simulink model "KD_cl_harness_forthao"  (R2015a)
settings: Solver=ode45  StartTime=0  StopTime=50  FixedStep=0.01  MaxStep=0.005  RelTol=1e-4  AbsTol=1e-4
InitFcn:
  | load KD_const_coeffs_0624
  | load pexhat_stuff
  | load expcon
  | load thr_ff_map
values from neighbouring files (symbols this model uses):
  c_0 = 0    [expcon.mat]
  c_1 = 1    [expcon.mat]
  c_100 = 100    [expcon.mat]
  c_1000 = 1000    [expcon.mat]
  c_10000 = 10000    [expcon.mat]
  c_1000inv = 0.0010000000475    [expcon.mat]    (also in pexhat_stuff.mat)
  c_100inv = 0.00999999977648    [expcon.mat]
  c_1_int = 1    [expcon.mat]
  c_1d2p4 = 0.416666656733    [expcon.mat]
  c_1p7 = 1.70000004768    [expcon.mat]
  c_4400inv = 0.000227272728807    [pexhat_stuff.mat]
  c_5500inv = 0.000181818177225    [expcon.mat]
  c_80 = 80    [expcon.mat]
  c_90 = 90    [expcon.mat]
  c_cal_phi = 7.6395999713e-06    [expcon.mat]
  c_compmap = [28125.0058594 29577.4082031 31350.1035156 33776.21875 37051.9296875 41026.2695312 45453.9960938 50160.3515625 55029.671875 59986.109375 64980.4296875 69980.4375 ... (320 elements, 20x16)]    [expcon.mat]
  c_ctok = 273.149993896    [expcon.mat]
  c_fflow_max = inf    [expcon.mat]
  c_fflow_min = 0    [expcon.mat]
  c_filt = 0.949999988079    [expcon.mat]
  c_flowdiv = 9.99999974738e-05    [expcon.mat]
  c_flowmin = 0    [expcon.mat]
  c_flowmult = 10000    [expcon.mat]
  c_inf = inf    [expcon.mat]
  c_km1d2k = 0.142857149243    [expcon.mat]
  c_mm3tokgpers = 2.77333338516e-08    [expcon.mat]
  c_n1 = -1    [expcon.mat]
  c_p00001 = 9.99999974738e-06    [expcon.mat]
  c_p01 = 0.00999999977648    [pexhat_stuff.mat]
  c_p016 = 0.01600000076    [expcon.mat]
  c_p1429 = 0.142900004983    [expcon.mat]
  c_p1e9 = 9.99999971718e-10    [expcon.mat]
  c_p4167 = 0.416700005531    [expcon.mat]    (also in pexhat_stuff.mat = 0.416666656733)
  c_p4d1p4 = 0.285714298487    [expcon.mat]
  c_p5401 = 0.540099978447    [expcon.mat]
  c_p9 = 0.899999976158    [expcon.mat]
  c_pincomp = 97.4216003418    [expcon.mat]
  c_ra = 287.002807617    [expcon.mat]
  c_rair = 287.09979248    [expcon.mat]
  c_Rby1000 = 0.000287000002572    [expcon.mat]
  c_roacorr = 8.05689978733e-06    [expcon.mat]
  c_rpmtoradpers = 0.104719758034    [expcon.mat]
  c_svrthrottle1 = [0.924875080585 0.575991511345 0.0858279466629 0.820202827454 0.445821881294 0.509882986546 0.0428557097912 0.753634572029 0]    [expcon.mat]
  c_svrthrottle2 = [0.145454958081 0.14545533061 0.363636374474 0.509091556072 0.509090721607 0.509091317654 0.545454084873 0.618182241917 0.145454272628]    [expcon.mat]
  c_svrthrottlearg = 0.10000000149    [expcon.mat]
  c_svrthrottlebeta = [2282.12670898 -3239.46044922 -142.784469604 -2660.34570312 1434.34350586 4150.43994141 -1580.68164062 -1039.89575195 791.34588623]    [expcon.mat]
  c_ta_max = inf    [expcon.mat]
  c_ta_min = 270    [expcon.mat]
  c_V = 0.0077999997884    [expcon.mat]
  c_vnliftmax = 90    [expcon.mat]
  c_vnliftmin = 40    [expcon.mat]
  Coefs =     [KD_const_coeffs_0624.mat]    (also in pexhat_stuff.mat)
  const =     [KD_const_coeffs_0624.mat]    (also in pexhat_stuff.mat)
  const_exhat =     [pexhat_stuff.mat]
  eegr_map =     [expcon.mat]
  egrr_delay_init = 0    [expcon.mat]
  epim_map =     [expcon.mat]
  eplufin_ff_map =     [expcon.mat]
  expcon =     [expcon.mat]
  invta = [5 5 5 5 2.5 0 0 0 0 0 0 0 ... (240 elements, 16x15)]    [expcon.mat]
  invtacols = [1000 1200 1400 1600 1800 2000 2200 2400 2600 2800 3000 3200 ... (16 elements, 1x16)]    [expcon.mat]
  IV =     [KD_const_coeffs_0624.mat]    (also in pexhat_stuff.mat)
  Lobs_init = [0 0 0]    [expcon.mat]
  map_delay_init = 120    [expcon.mat]
  maxA_t = [51.4567184448 53.8593139648 56.3063011169 58.7576789856 61.1701469421 63.4982337952 65.6955718994 67.7161483765 69.5156555176 71.0527648926 72.2902603149 73.1961746216 ... (16 elements, 1x16)]    [expcon.mat]
  obsA = [0.985195398331  0  0; -0.188821405172  1  0; 0.000342977960827  0  1]    [expcon.mat]
  sample_time = 0.016    [expcon.mat]    (also in pexhat_stuff.mat)
  SVR_EGR =     [KD_const_coeffs_0624.mat]    (also in pexhat_stuff.mat)
  SVR_EGR_exhat =     [pexhat_stuff.mat]
  SVR_throttle =     [KD_const_coeffs_0624.mat]    (also in pexhat_stuff.mat)
  uz_init = [0 0]    [expcon.mat]
undefined symbols (not defined in the file or in its folder): k1_table, k2_table, maxL, minL, Newton, Raphson
libraries: simulink x5
(part 1 of 6)
settings Model: CovSFcnEnable=off  Creator=spolavarapu  LastModifiedBy=258242
settings SolverCC: ZeroCrossControl=DisableAll
settings DataIOCC: LimitDataPoints=off  SaveFormat=StructureWithTime  SignalLoggingSaveFormat=ModelDataLogs  SaveState=on  DSMLogging=off
settings OptimizationCC: BlockReduction=off  OptimizeBlockIOStorage=off  BufferReuse=off  GlobalBufferReuse=off  ExpressionFolding=off  ExpressionDepthLimit=2147483647  LocalBlockOutputs=off  EfficientFloat2IntCast=on  OptimizeModelRefInitCode=on
settings DebuggingCC: SignalInfNanChecking=error  SignalRangeChecking=error  ReadBeforeWriteMsg=DisableAll  WriteAfterWriteMsg=DisableAll  WriteAfterReadMsg=DisableAll  AlgebraicLoopMsg=error  ArtificialAlgebraicLoopMsg=error  SaveWithDisabledLinksMsg=error  SaveWithParameterizedLinksMsg=error  UnderspecifiedInitializationDetection=Classic  MergeDetectMultiDrivingBlocksExec=none  CheckExecutionContextPreStartOutputMsg=on  CheckExecutionContextRuntimeOutputMsg=on  BlockPriorityViolationMsg=error  SolverPrmCheckMsg=error  InheritedTsInSrcMsg=error  DiscreteInheritContinuousMsg=error  MultiTaskDSMMsg=none  SigSpecEnsureSampleTimeMsg=error  CheckMatrixSingularityMsg=error  IntegerOverflowMsg=error  ParameterUnderflowMsg=error  ParameterPrecisionLossMsg=error  ParameterTunabilityLossMsg=error  UnderSpecifiedDataTypeMsg=warning  UnnecessaryDatatypeConvMsg=warning  VectorMatrixConversionMsg=error  FcnCallInpInsideContextMsg=EnableAllAsWarning  SignalLabelMismatchMsg=warning  UnconnectedInputMsg=error  UnconnectedOutputMsg=error  UnconnectedLineMsg=error  SFcnCompatibilityMsg=error  UniqueDataStoreMsg=error  BusObjectLabelMismatch=error  RootOutportRequireBusObject=error  AssertControl=DisableAll  ModelReferenceIOMsg=error  ModelReferenceIOMismatchMessage=error  UnknownTsInhSupMsg=error  ModelReferenceDataLoggingMessage=error  StateNameClashWarn=warning  StrictBusMsg=ErrorOnBusTreatedAsVector  IntegerSaturationMsg=error
settings RTWCC: SystemTargetFile=ert.tlc  TemplateMakefile=ert_default_tmf  Description=Real-Time Workshop Embedded Coder
settings CodeAppCC: ForceParamTrailComments=on  IgnoreCustomStorageClasses=off  MangleLength=4  CustomSymbolStrType=$N$R$M  InternalIdentifier=Classic  ReqsInCode=on
settings ERTTargetCC: ParMdlRefBuildCompliant=on  CompOptLevelCompliant=on  ConcurrentExecutionCompliant=on  IncludeMdlTerminateFcn=off  GeneratePreprocessorConditionals=Disable all  SuppressErrorStatus=on  ERTFirstTimeCompliant=on  SupportAbsoluteTime=off  SupportNonFinite=off  SupportContinuousTime=off  SupportVariableSizeSignals=off  ParenthesesLevel=Maximum  ModelStepFunctionPrototypeControlCompliant=on  CPPClassGenCompliant=on  InlinedParameterPlacement=Hierarchical  ERTCustomFileTemplate=example_file_process.tlc  PreserveExpressionOrder=on  PreserveIfCondition=on

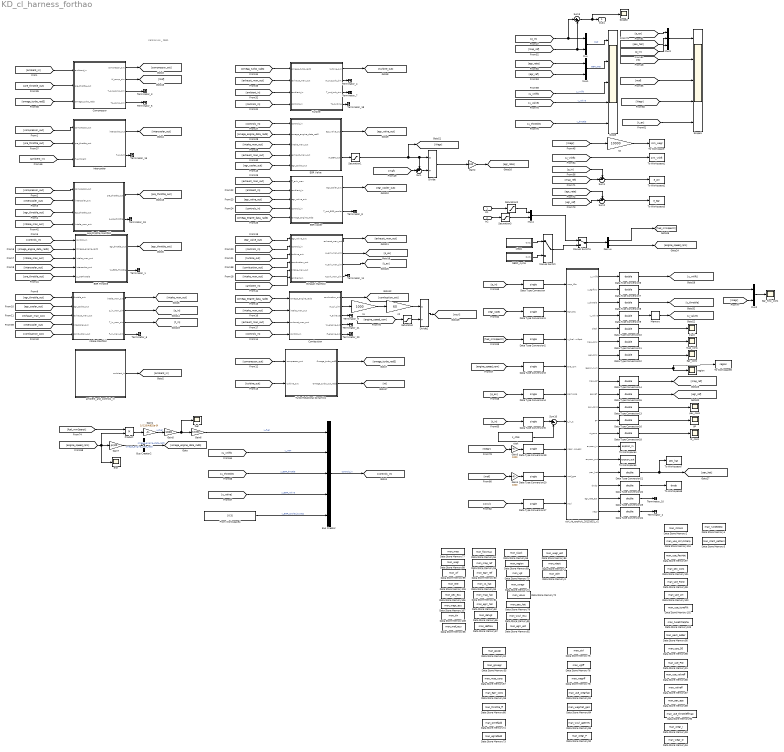
== system KD_cl_harness_forthao ==
  note: Version A4 _ 0611
  In1 : Inport  Interpolate=off
  In2 : Inport  Port=2  Interpolate=off
  Bus Creator : BusCreator  Inputs=5
  Bus Creator2 : BusCreator  Inputs=1
  Combsution : Subsystem
  Compressor : Subsystem
  Data Store Memory1 : DataStoreMemory  DataStoreName=mon_ntest  ReadBeforeWriteMsg=warning  WriteAfterWriteMsg=warning  WriteAfterReadMsg=warning  OutDataTypeStr=single
  Data Store Memory100 : DataStoreMemory  DataStoreName=man_use_LM  ReadBeforeWriteMsg=warning  WriteAfterWriteMsg=warning  WriteAfterReadMsg=warning  InitialValue=1  OutDataTypeStr=single
  Data Store Memory101 : DataStoreMemory  DataStoreName=man_pex_cons  ReadBeforeWriteMsg=warning  WriteAfterWriteMsg=warning  WriteAfterReadMsg=warning  InitialValue=200  OutDataTypeStr=single
  Data Store Memory102 : DataStoreMemory  DataStoreName=man_use_tuneFilt  ReadBeforeWriteMsg=warning  WriteAfterWriteMsg=warning  WriteAfterReadMsg=warning  InitialValue=1  OutDataTypeStr=single
  Data Store Memory103 : DataStoreMemory  DataStoreName=man_tuneFiltalpha  ReadBeforeWriteMsg=warning  WriteAfterWriteMsg=warning  WriteAfterReadMsg=warning  InitialValue=single(.9)  OutDataTypeStr=single
  Data Store Memory104 : DataStoreMemory  DataStoreName=man_use_Wcylinterp  ReadBeforeWriteMsg=warning  WriteAfterWriteMsg=warning  WriteAfterReadMsg=warning  OutDataTypeStr=single
  Data Store Memory105 : DataStoreMemory  DataStoreName=mon_ene  ReadBeforeWriteMsg=warning  WriteAfterWriteMsg=warning  WriteAfterReadMsg=warning  InitialValue=1  OutDataTypeStr=single
  Data Store Memory106 : DataStoreMemory  DataStoreName=mon_pex_ecu  ReadBeforeWriteMsg=warning  WriteAfterWriteMsg=warning  WriteAfterReadMsg=warning  InitialValue=1  OutDataTypeStr=single
  Data Store Memory107 : DataStoreMemory  DataStoreName=mon_wegr_ecu  ReadBeforeWriteMsg=warning  WriteAfterWriteMsg=warning  WriteAfterReadMsg=warning  InitialValue=1  OutDataTypeStr=single
  Data Store Memory108 : DataStoreMemory  DataStoreName=mon_tin  ReadBeforeWriteMsg=warning  WriteAfterWriteMsg=warning  WriteAfterReadMsg=warning  InitialValue=1  OutDataTypeStr=single
  Data Store Memory2 : DataStoreMemory  DataStoreName=man_ntcons  ReadBeforeWriteMsg=warning  WriteAfterWriteMsg=warning  WriteAfterReadMsg=warning  InitialValue=13000  OutDataTypeStr=single
  Data Store Memory3 : DataStoreMemory  DataStoreName=mon_pthr  ReadBeforeWriteMsg=warning  WriteAfterWriteMsg=warning  WriteAfterReadMsg=warning  OutDataTypeStr=single
  Data Store Memory4 : DataStoreMemory  DataStoreName=man_run2500tp  ReadBeforeWriteMsg=warning  WriteAfterWriteMsg=warning  WriteAfterReadMsg=warning  OutDataTypeStr=single
  Data Store Memory5 : DataStoreMemory  DataStoreName=man_start_pattern  ReadBeforeWriteMsg=warning  WriteAfterWriteMsg=warning  WriteAfterReadMsg=warning  InitialValue=1  OutDataTypeStr=single
  Data Store Memory52 : DataStoreMemory  DataStoreName=man_gsvgt  ReadBeforeWriteMsg=warning  WriteAfterWriteMsg=warning  WriteAfterReadMsg=warning  InitialValue=1  OutDataTypeStr=single
  Data Store Memory55 : DataStoreMemory  DataStoreName=man_gswegr  ReadBeforeWriteMsg=warning  WriteAfterWriteMsg=warning  WriteAfterReadMsg=warning  InitialValue=1  OutDataTypeStr=single
  Data Store Memory56 : DataStoreMemory  DataStoreName=mon_maf_ecu  ReadBeforeWriteMsg=warning  WriteAfterWriteMsg=warning  WriteAfterReadMsg=warning  InitialValue=1  OutDataTypeStr=single
  Data Store Memory57 : DataStoreMemory  DataStoreName=man_map_cons  ReadBeforeWriteMsg=warning  WriteAfterWriteMsg=warning  WriteAfterReadMsg=warning  InitialValue=165  OutDataTypeStr=single
  Data Store Memory58 : DataStoreMemory  DataStoreName=man_egrr_cons  ReadBeforeWriteMsg=warning  WriteAfterWriteMsg=warning  WriteAfterReadMsg=warning  InitialValue=40  OutDataTypeStr=single
  Data Store Memory59 : DataStoreMemory  DataStoreName=mon_map_ref  ReadBeforeWriteMsg=warning  WriteAfterWriteMsg=warning  WriteAfterReadMsg=warning  InitialValue=1  OutDataTypeStr=single
  Data Store Memory60 : DataStoreMemory  DataStoreName=mon_egrr_ref  ReadBeforeWriteMsg=warning  WriteAfterWriteMsg=warning  WriteAfterReadMsg=warning  InitialValue=1  OutDataTypeStr=single
  Data Store Memory61 : DataStoreMemory  DataStoreName=mon_map_hat  ReadBeforeWriteMsg=warning  WriteAfterWriteMsg=warning  WriteAfterReadMsg=warning  InitialValue=1  OutDataTypeStr=single
  Data Store Memory62 : DataStoreMemory  DataStoreName=mon_egrr_hat  ReadBeforeWriteMsg=warning  WriteAfterWriteMsg=warning  WriteAfterReadMsg=warning  InitialValue=1  OutDataTypeStr=single
  Data Store Memory63 : DataStoreMemory  DataStoreName=mon_x1_hat  ReadBeforeWriteMsg=warning  WriteAfterWriteMsg=warning  WriteAfterReadMsg=warning  InitialValue=1  OutDataTypeStr=single
  Data Store Memory64 : DataStoreMemory  DataStoreName=mon_flowmax  ReadBeforeWriteMsg=warning  WriteAfterWriteMsg=warning  WriteAfterReadMsg=warning  InitialValue=1  OutDataTypeStr=single
  Data Store Memory65 : DataStoreMemory  DataStoreName=mon_delvgt  ReadBeforeWriteMsg=warning  WriteAfterWriteMsg=warning  WriteAfterReadMsg=warning  InitialValue=1  OutDataTypeStr=single
  Data Store Memory66 : DataStoreMemory  DataStoreName=man_throttle_ff  ReadBeforeWriteMsg=warning  WriteAfterWriteMsg=warning  WriteAfterReadMsg=warning  OutDataTypeStr=single
  Data Store Memory67 : DataStoreMemory  DataStoreName=mon_delflow  ReadBeforeWriteMsg=warning  WriteAfterWriteMsg=warning  WriteAfterReadMsg=warning  InitialValue=1  OutDataTypeStr=single
  Data Store Memory68 : DataStoreMemory  DataStoreName=mon_slack  ReadBeforeWriteMsg=warning  WriteAfterWriteMsg=warning  WriteAfterReadMsg=warning  InitialValue=1  OutDataTypeStr=single
  Data Store Memory69 : DataStoreMemory  DataStoreName=mon_region  ReadBeforeWriteMsg=warning  WriteAfterWriteMsg=warning  WriteAfterReadMsg=warning  InitialValue=1  OutDataTypeStr=int32
  Data Store Memory70 : DataStoreMemory  DataStoreName=mon_vgt  ReadBeforeWriteMsg=warning  WriteAfterWriteMsg=warning  WriteAfterReadMsg=warning  InitialValue=1  OutDataTypeStr=single
  Data Store Memory71 : DataStoreMemory  DataStoreName=mon_uwegr  ReadBeforeWriteMsg=warning  WriteAfterWriteMsg=warning  WriteAfterReadMsg=warning  InitialValue=1  OutDataTypeStr=single
  Data Store Memory72 : DataStoreMemory  DataStoreName=mon_valve  ReadBeforeWriteMsg=warning  WriteAfterWriteMsg=warning  WriteAfterReadMsg=warning  InitialValue=1  OutDataTypeStr=single
  Data Store Memory73 : DataStoreMemory  DataStoreName=man_egrrefadd  ReadBeforeWriteMsg=warning  WriteAfterWriteMsg=warning  WriteAfterReadMsg=warning  InitialValue=-35  OutDataTypeStr=single
  Data Store Memory74 : DataStoreMemory  DataStoreName=man_pinrefadd  ReadBeforeWriteMsg=warning  WriteAfterWriteMsg=warning  WriteAfterReadMsg=warning  InitialValue=c_pinrefadd  OutDataTypeStr=single
  Data Store Memory75 : DataStoreMemory  DataStoreName=man_ctrl  ReadBeforeWriteMsg=warning  WriteAfterWriteMsg=warning  WriteAfterReadMsg=warning  OutDataTypeStr=single
  Data Store Memory76 : DataStoreMemory  DataStoreName=man_vgtff  ReadBeforeWriteMsg=warning  WriteAfterWriteMsg=warning  WriteAfterReadMsg=warning  InitialValue=70  OutDataTypeStr=single
  Data Store Memory77 : DataStoreMemory  DataStoreName=mon_map  ReadBeforeWriteMsg=warning  WriteAfterWriteMsg=warning  WriteAfterReadMsg=warning  InitialValue=1  OutDataTypeStr=single
  Data Store Memory78 : DataStoreMemory  DataStoreName=man_wegrff  ReadBeforeWriteMsg=warning  WriteAfterWriteMsg=warning  WriteAfterReadMsg=warning  InitialValue=3  OutDataTypeStr=single
  Data Store Memory79 : DataStoreMemory  DataStoreName=mon_pex_hat  ReadBeforeWriteMsg=warning  WriteAfterWriteMsg=warning  WriteAfterReadMsg=warning  InitialValue=3  OutDataTypeStr=single
  Data Store Memory80 : DataStoreMemory  DataStoreName=mon_wcyl_ecu  ReadBeforeWriteMsg=warning  WriteAfterWriteMsg=warning  WriteAfterReadMsg=warning  InitialValue=1  OutDataTypeStr=single
  Data Store Memory81 : DataStoreMemory  DataStoreName=man_use_wegrhat  ReadBeforeWriteMsg=warning  WriteAfterWriteMsg=warning  WriteAfterReadMsg=warning  InitialValue=1  OutDataTypeStr=single
  Data Store Memory82 : DataStoreMemory  DataStoreName=mon_egrr_est  ReadBeforeWriteMsg=warning  WriteAfterWriteMsg=warning  WriteAfterReadMsg=warning  InitialValue=1  OutDataTypeStr=single
  Data Store Memory83 : DataStoreMemory  DataStoreName=mon_wegr_est  ReadBeforeWriteMsg=warning  WriteAfterWriteMsg=warning  WriteAfterReadMsg=warning  InitialValue=1  OutDataTypeStr=single
  Data Store Memory84 : DataStoreMemory  DataStoreName=man_wegrhat_gain  ReadBeforeWriteMsg=warning  WriteAfterWriteMsg=warning  WriteAfterReadMsg=warning  InitialValue=350  OutDataTypeStr=single
  Data Store Memory85 : DataStoreMemory  DataStoreName=man_wcyl_gperrev  ReadBeforeWriteMsg=warning  WriteAfterWriteMsg=warning  WriteAfterReadMsg=warning  InitialValue=1  OutDataTypeStr=single
  Data Store Memory86 : DataStoreMemory  DataStoreName=man_use_valveff  ReadBeforeWriteMsg=warning  WriteAfterWriteMsg=warning  WriteAfterReadMsg=warning  OutDataTypeStr=single
  Data Store Memory87 : DataStoreMemory  DataStoreName=man_valveff  ReadBeforeWriteMsg=warning  WriteAfterWriteMsg=warning  WriteAfterReadMsg=warning  OutDataTypeStr=single
  Data Store Memory88 : DataStoreMemory  DataStoreName=mon_wegr  ReadBeforeWriteMsg=warning  WriteAfterWriteMsg=warning  WriteAfterReadMsg=warning  InitialValue=1  OutDataTypeStr=single
  Data Store Memory89 : DataStoreMemory  DataStoreName=man_pex_eps  ReadBeforeWriteMsg=warning  WriteAfterWriteMsg=warning  WriteAfterReadMsg=warning  InitialValue=single(.0000001)  OutDataTypeStr=single
  Data Store Memory90 : DataStoreMemory  DataStoreName=man_use_throttleffmap  ReadBeforeWriteMsg=warning  WriteAfterWriteMsg=warning  WriteAfterReadMsg=warning  OutDataTypeStr=single
  Data Store Memory91 : DataStoreMemory  DataStoreName=man_use_PID  ReadBeforeWriteMsg=warning  WriteAfterWriteMsg=warning  WriteAfterReadMsg=warning  OutDataTypeStr=single
  Data Store Memory92 : DataStoreMemory  DataStoreName=man_wegr_P  ReadBeforeWriteMsg=warning  WriteAfterWriteMsg=warning  WriteAfterReadMsg=warning  InitialValue=1  OutDataTypeStr=single
  Data Store Memory93 : DataStoreMemory  DataStoreName=man_wegr_I  ReadBeforeWriteMsg=warning  WriteAfterWriteMsg=warning  WriteAfterReadMsg=warning  InitialValue=.0625  OutDataTypeStr=single
  Data Store Memory94 : DataStoreMemory  DataStoreName=man_wegr_D  ReadBeforeWriteMsg=warning  WriteAfterWriteMsg=warning  WriteAfterReadMsg=warning  OutDataTypeStr=single
  Data Store Memory95 : DataStoreMemory  DataStoreName=man_pexh_adder  ReadBeforeWriteMsg=warning  WriteAfterWriteMsg=warning  WriteAfterReadMsg=warning  OutDataTypeStr=single
  Data Store Memory96 : DataStoreMemory  DataStoreName=man_use_SG  ReadBeforeWriteMsg=warning  WriteAfterWriteMsg=warning  WriteAfterReadMsg=warning  OutDataTypeStr=single
  Data Store Memory97 : DataStoreMemory  DataStoreName=man_use_PexHat  ReadBeforeWriteMsg=warning  WriteAfterWriteMsg=warning  WriteAfterReadMsg=warning  InitialValue=1  OutDataTypeStr=single
  Data Store Memory98 : DataStoreMemory  DataStoreName=man_use_ROO  ReadBeforeWriteMsg=warning  WriteAfterWriteMsg=warning  WriteAfterReadMsg=warning  InitialValue=1  OutDataTypeStr=single
  Data Store Memory99 : DataStoreMemory  DataStoreName=mon_wf  ReadBeforeWriteMsg=warning  WriteAfterWriteMsg=warning  WriteAfterReadMsg=warning  InitialValue=1  OutDataTypeStr=single
  Data Type Conversion{,1..5,17,19..20} (9 alike) : DataTypeConversion  OutDataTypeStr=single
  Data Type Conversion{6..16,18,21..24} (16 alike) : DataTypeConversion  OutDataTypeStr=double
  Demux : Demux  Outputs=2
  Divide : Product  Inputs=*/
  Divide1 : Product  Inputs=*/
  EGR Throttle : Subsystem
  EGR Valve : Subsystem
  EGR cooler : Subsystem
  Exhaust Manifold : Subsystem
  From Workspace4 : FromWorkspace  VariableName=[0 3]  SampleTime=0  Interpolate=off  OutputAfterFinalValue=Holding final value
  Gain1 : Gain  Gain=1/(120/4/832e-9)
  Gain2 : Gain  Gain=100
  Gain3 : Gain  Gain=1000
  Gain4 : Gain  Gain=1000
  Gain5 : Gain  Gain=1000
  Gain6 : Gain  Gain=1/1000
  Gain7 : Gain  Gain=pi/30
  Intake Manifold : Subsystem
  Intercooler : Subsystem
  Manual Switch : ManualSwitch
  Manual Switch1 : ManualSwitch
  Memory : Memory
  Mux{,1..2,4} (4 alike) : Mux  Inputs=2
  Mux3 : Mux  Inputs=3
  NEDC_cycle : Subsystem
  Product : Product  RndMeth=Zero
  Saturation : Saturate  UpperLimit=6000  LowerLimit=500
  Saturation1 : Saturate  UpperLimit=inf  LowerLimit=0
      settings: AttributesFormatString=%<LowerLimit>\n%<UpperLimit>
  Saturation2 : Saturate  UpperLimit=45  LowerLimit=5
  Saturation3 : Saturate  UpperLimit=3000  LowerLimit=1800
  Scope : Scope  NumInputPorts=5
      settings: TimeRange=1  YMin=0~-1~48.506~4.75~-1  YMax=110~1~53.6118~5.25~1  SaveName=scope
  Scope1 : Scope  NumInputPorts=5
      settings: TimeRange=5  YMin=0~1800~0~0~400  YMax=600~2200~0.015~0.004~600
  Scope2 : Scope
      settings: YMin=-40  YMax=15
  Sum : Sum  Inputs=++|
  Sum1 : Sum  Inputs=+-|
  Sum10 : Sum  Inputs=|+-
  Sum2 : Sum  Inputs=+-|
  Sum3 : Sum  Inputs=|+-
  Terminator_{1..11,15,18..21} (16 alike) : Terminator
  To Workspace : ToWorkspace  VariableName=sim_wegr  SampleTime=-1
  To Workspace1 : ToWorkspace  VariableName=sim_vnlift  SampleTime=-1
  To Workspace2 : ToWorkspace  VariableName=e_pin  SampleTime=-1
  To Workspace3 : ToWorkspace  VariableName=e_egr  SampleTime=-1
  To Workspace4 : ToWorkspace  VariableName=expcon_in  SaveFormat=Structure  SampleTime=-1
  To Workspace5 : ToWorkspace  VariableName=expcon_out  SaveFormat=Structure  SampleTime=-1
  To Workspace6 : ToWorkspace  VariableName=region  SaveFormat=Structure With Time  SampleTime=-1
  To Workspace7 : ToWorkspace  VariableName=pex_hat  SaveFormat=Structure With Time  SampleTime=-1
  To Workspace8 : ToWorkspace  VariableName=dwdp  SaveFormat=Structure With Time  SampleTime=-1
  Turbine : Subsystem
  Turbo Rotational Dynamics : Subsystem
  ambient_and_controls_in : Subsystem
  ctok : Constant  Value=c_ctok  OutDataTypeStr=single  SampleTime=sample_time
      settings: AttributesFormatString=%<Value>\n%<SampleTime>
  ctrl_rb_explicit_20131031_v2 : Subsystem  TreatAsAtomicUnit=on  SystemSampleTime=sample_time
  egr_cons : Scope
      settings: TimeRange=30  YMin=0  YMax=40  SaveName=egr_cons  SampleTime=.032
  egr_flow_cons : Scope
      settings: YMin=0  YMax=0.0045  SaveName=egr_flow_cons  SampleTime=.032
  ene : Scope
      settings: YMin=2000  YMax=2250  SaveName=ene_rpm  SampleTime=.032
  fuel : Scope
      settings: YMin=2.5  YMax=30  SaveName=fuel_gpers  SampleTime=.032
  gs : Scope
      settings: TimeRange=30  YMin=0.5  YMax=5.25  SaveName=gs  SampleTime=.032
  map_cons : Scope
      settings: TimeRange=30  YMin=90  YMax=300  SaveName=map_cons  SampleTime=.032
  n1 : Gain  Gain=1000
      settings: AttributesFormatString=%<Gain>
  n2 : Gain  Gain=60
      settings: AttributesFormatString=%<Gain>
  n3 : Gain  Gain=10000
      settings: AttributesFormatString=%<Gain>
  nt_cons : Scope
      settings: TimeRange=30  YMin=1.5  YMax=12.5  SaveName=nt_cons  SampleTime=.032
  pex_cons : Scope
      settings: TimeRange=30  YMin=100  YMax=400  SaveName=pex_cons  SampleTime=.032
  pre-throttle manifold : Subsystem
  region : Scope
      settings: TimeRange=100  YMin=-1  YMax=1  SaveName=outs  SampleTime=.032
  slack : Scope
      settings: YMin=-1  YMax=1  SaveName=outs1  SampleTime=.032
  steps : Subsystem
  Out1 : Outport
  wires:
  ambient_and_controls_in/1(ambient_in) -> [ambient_in]
  Compressor/1(compressor_out) -> [compressor_out]
  Intercooler/1(intercooler_out) -> [intercooler_out]
  EGR Throttle/1(egr_throttle_out) -> [egr_throttle_out]
  Intake Manifold/1(intake_man_out) -> [intake_man_out]
  Turbine/1(turbine_out) -> [turbine_out]
  EGR Valve/1(egr_valve_out) -> [egr_valve_out]
  EGR cooler/1(egr_cooler_out) -> [egr_cooler_out]
  Exhaust Manifold/1(exhaust_man_out) -> [exhaust_man_out]
  Combsution/1(combustion_out) -> [combustion_out]
  pre-throttle manifold/1(pre_throttle_out) -> [pre_throttle_out]
  Compressor/2(W_comp_sim) -> [maf]
  Compressor/3(T_out_comp_sim) -> Terminator_3/1
  Compressor/4(Tq_comp_sim) -> Terminator_5/1
  EGR Valve/2(W_EGR_out) -> Saturation1/1
  Exhaust Manifold/4(F_exh_man_sim) -> Terminator_11/1
  Intake Manifold/3(T_in_man_sim) -> [t_in]
  Intercooler/2(T_out_IC) -> Terminator_15/1
  Turbine/4(Tq_turbine) -> Terminator_18/1
  pre-throttle manifold/2(p_pre_throttle) -> Terminator_19/1
  Turbo Rotational Dynamics/1(Omega_turbo_radS) -> [omega_turbo_radS]
  Combsution/4(W_engine_out) -> Terminator_21/1
  Combsution/5(F_engine_out) -> Terminator_20/1
  Intake Manifold/2(p_in_man_sim) -> [p_in]
  Turbo Rotational Dynamics/2(Omega_turbo_out_radS) -> [nt]
  [maf] -> Sum/2
  Sum/1 -> Divide/2
  Divide/1 -> Gain2/1
  Exhaust Manifold/2(p_exh_man_sim) -> [p_ex]
  Turbine/2(W_out_turb_sim) -> Terminator_4/1
  Turbine/3(T_out_turb_sim) -> Terminator_7/1
  [p_in] -> Sum3/1, Mux/1
  [egr_rate] -> Mux1/1
  [u_vnlift] -> Bus Creator/2  "u_VGT"
  [u_throttle] -> Bus Creator/3  "u_EGR_throttle"
  [u_valve] -> Bus Creator/4  "u_EGR_valve"
  From Workspace4/1 -> Bus Creator/5  "u_EGR_cooler_bypass"
  Bus Creator/1 -> [controls_in]  "controls_in"
  Bus Creator2/1 -> [omega_engine_data_radS]  "omega_engine_data_radS"
  Mux/1 -> Scope/1  "MAP"
  Mux1/1 -> Scope/2  "EGR_rate"
  [map_ref] -> Mux/2, Sum3/2
  [egr_ref] -> Mux1/2
  Gain2/1 -> [egr_rate]
  Exhaust Manifold/3(T_exh_man_sim) -> [t_ex]
  ctrl_rb_explicit_20131031_v2/3(u_throttle) -> Data Type Conversion8/1
  ctrl_rb_explicit_20131031_v2/2(u_egrflow) -> Data Type Conversion7/1
  ctrl_rb_explicit_20131031_v2/4(u_valve) -> Data Type Conversion9/1
  ctrl_rb_explicit_20131031_v2/5(slack) -> Data Type Conversion10/1
  ctrl_rb_explicit_20131031_v2/6(map_cons) -> Data Type Conversion11/1
  ctrl_rb_explicit_20131031_v2/7(egr_cons) -> Data Type Conversion12/1
  Gain7/1 -> Bus Creator2/1  "omega_engine_data_radS"
  [engine_speed_rpm] -> Gain7/1, Product/2, ene/1
  ctrl_rb_explicit_20131031_v2/1(u_vnlift) -> Data Type Conversion6/1
  [p_in] -> Data Type Conversion/1
  [egr_rate] -> Data Type Conversion1/1
  [fuel_mm3perst] -> Data Type Conversion2/1
  [engine_speed_rpm] -> Data Type Conversion3/1
  [p_ex] -> Data Type Conversion4/1
  [t_in] -> Data Type Conversion5/1
  ctrl_rb_explicit_20131031_v2/8(region_num) -> region/1, To Workspace6/1
  ctrl_rb_explicit_20131031_v2/9(map_ref) -> Data Type Conversion14/1
  ctrl_rb_explicit_20131031_v2/10(egr_ref) -> Data Type Conversion15/1
  Data Type Conversion6/1 -> [u_vnlift]
  Data Type Conversion8/1 -> [u_throttle]
  Data Type Conversion9/1 -> Memory/1
  Data Type Conversion10/1 -> slack/1
  Data Type Conversion11/1 -> map_cons/1
  Data Type Conversion12/1 -> egr_cons/1
  Data Type Conversion14/1 -> [map_ref]
  Data Type Conversion15/1 -> [egr_ref]
  [nt] -> Scope1/2
  [maf] -> Scope1/3
  [Wegr] -> Scope1/4
  [t_ex] -> Scope1/5
  [u_vnlift] -> Scope/3  "u_vnlift"
  [u_valve] -> Scope/4  "u_valve"
  EGR Throttle/2(W_EGR_Throttle) -> Terminator_1/1
  Saturation1/1 -> Sum/1, Divide/1, [Wegr]
  [ambient_in] -> Compressor/1(ambient_in)
  [compressor_out] -> Intercooler/1(compressor_out)
  [compressor_out] -> pre-throttle manifold/1(compressor_out)
  [intercooler_out] -> pre-throttle manifold/2(intercooler_out)
  [egr_throttle_out] -> pre-throttle manifold/3(egr_throttle_out)
  [controls_in] -> EGR Throttle/1(controls_in)
  [omega_engine_data_radS] -> EGR Throttle/2(Omega_engine_radS)
  [intake_man_out] -> EGR Throttle/3(intake_man_out)
  [intercooler_out] -> EGR Throttle/4(intercooler_out)
  [egr_throttle_out] -> Intake Manifold/1(throttle_out)
  [egr_cooler_out] -> Intake Manifold/2(egr_cooler_out)
  [exhaust_man_out] -> Intake Manifold/3(exhaust_man_out)
  [omega_turbo_radS] -> Compressor/3(Omega_turbo_radS)
  [pre_throttle_out] -> Compressor/2(pre_throttle_out)
  [pre_throttle_out] -> Intercooler/2(pre_throttle_out)
  [intercooler_out] -> Intake Manifold/4(intecooler_out)
  [combustion_out] -> Intake Manifold/5(combustion_out)
  [pre_throttle_out] -> EGR Throttle/5(p_preThrottle)
  [intake_man_out] -> pre-throttle manifold/4(Intake_man_out)
  [ambient_in] -> Intercooler/3(T_ambient)
  [omega_engine_data_radS] -> Combsution/1(Omega_engine_radS)
  [intake_man_out] -> Combsution/2(intake_man_out)
  [exhaust_man_out] -> Combsution/3(exhaust_man_out)
  [controls_in] -> Combsution/4(controls_in)
  [intake_man_out] -> Exhaust Manifold/5(intake_man_out)
  [egr_valve_out] -> Exhaust Manifold/1(egr_valve_out)
  [controls_in] -> Exhaust Manifold/2(controls_in)
  [turbine_out] -> Exhaust Manifold/3(turbine_out)
  [ambient_in] -> EGR cooler/2(ambient_in)
  [exhaust_man_out] -> EGR cooler/1(T_exh_man)
  [egr_valve_out] -> EGR cooler/3(egr_valve_out)
  [controls_in] -> EGR cooler/4(controls_in)
  [omega_engine_data_radS] -> EGR cooler/5(Omega_engine_radS)
  [exhaust_man_out] -> EGR Valve/4(exhaust_man_out)
  [controls_in] -> EGR Valve/1(controls_in)
  [omega_engine_data_radS] -> EGR Valve/2(omega_engine_data_radS)
  [intake_man_out] -> EGR Valve/3(intake_man_out)
  [omega_turbo_radS] -> Turbine/1(omega_turbo_radS)
  [exhaust_man_out] -> Turbine/2(exhaust_man_out)
  [ambient_in] -> Turbine/3(ambient_In)
  [controls_in] -> Turbine/4(controls_In)
  [compressor_out] -> Turbo Rotational Dynamics/1(compressor_out)
  [turbine_out] -> Turbo Rotational Dynamics/2(turbine_out)
  [combustion_out] -> Exhaust Manifold/4(combustion_out)
  [egr_cooler_out] -> EGR Valve/5(egr_cooler_out)
  [ambient_in] -> Exhaust Manifold/6(ambient_in)
  Intake Manifold/4(F_in_man_sim) -> Terminator_6/1
  Combsution/3(T_exhaust) -> Terminator_9/1
  [Wegr] -> n3/1
  n3/1 -> To Workspace/1
  [u_vnlift] -> To Workspace1/1
  [map_ref] -> Sum1/2
  [p_in] -> Sum1/1
  Sum1/1 -> To Workspace2/1
  [egr_ref] -> Sum2/2
  [egr_rate] -> Sum2/1
  Sum2/1 -> To Workspace3/1
  Product/1 -> Gain1/1
  [fuel_mm3perst] -> Product/1
  [u_throttle] -> Scope/5  "u_throttle"
  NEDC_cycle/1(Out1) -> Manual Switch/2
  steps/1(Out1) -> Manual Switch/1
  Manual Switch/1 -> Manual Switch1/2
  ctrl_rb_explicit_20131031_v2/11(pex_cons) -> Data Type Conversion13/1
  Data Type Conversion13/1 -> pex_cons/1
  ctrl_rb_explicit_20131031_v2/12(gs) -> Data Type Conversion16/1
  Data Type Conversion16/1 -> gs/1
  Data Type Conversion18/1 -> nt_cons/1
  ctrl_rb_explicit_20131031_v2/13(nt_cons) -> Data Type Conversion18/1
  Data Type Conversion7/1 -> Mux2/1
  Mux2/1 -> egr_flow_cons/1
  [Wegr] -> Mux2/2
  ctrl_rb_explicit_20131031_v2/14(expcon_in) -> To Workspace4/1
  ctrl_rb_explicit_20131031_v2/15(expcon_out) -> To Workspace5/1
  Data Type Conversion/1 -> ctrl_rb_explicit_20131031_v2/1(map_kPa)
  Data Type Conversion1/1 -> ctrl_rb_explicit_20131031_v2/2(egrr_ecu)
  Data Type Conversion2/1 -> ctrl_rb_explicit_20131031_v2/3(u_fuel_mm3pst)
  Data Type Conversion3/1 -> ctrl_rb_explicit_20131031_v2/4(ene_rpm)
  Data Type Conversion4/1 -> ctrl_rb_explicit_20131031_v2/5(pexh_kpa)
  Memory/1 -> [u_valve]
  [Wegr] -> Gain3/1
  Gain3/1 -> Data Type Conversion19/1
  Data Type Conversion19/1 -> ctrl_rb_explicit_20131031_v2/7(wegrmeas_gps)
  ctrl_rb_explicit_20131031_v2/16(pex_hat) -> Data Type Conversion21/1
  [p_ex] -> Mux3/1
  Mux3/1 -> Scope1/1
  [pex_hat] -> Mux3/2
  Data Type Conversion21/1 -> To Workspace7/1, [pex_hat]
  Data Type Conversion22/1 -> To Workspace8/1
  ctrl_rb_explicit_20131031_v2/17(dwdp) -> Data Type Conversion22/1
  EGR cooler/2(T_out_EGR_cooler) -> Terminator_8/1
  Gain4/1 -> Data Type Conversion20/1
  [maf] -> Gain4/1
  Data Type Conversion20/1 -> ctrl_rb_explicit_20131031_v2/8(maf_gps)
  Gain5/1 -> fuel/1, Gain6/1
  Gain6/1 -> Bus Creator/1  "u_fuel"
  Gain1/1 -> Gain5/1  "u_fuel"
  [p_in] -> Mux3/3
  Data Type Conversion5/1 -> Sum10/1
  ctok/1 -> Sum10/2
  Sum10/1 -> ctrl_rb_explicit_20131031_v2/6(t_in_C)
  Combsution/2(W_cyl_sim) -> n1/1
  n1/1 -> n2/1
  n2/1 -> Divide1/1
  [engine_speed_rpm] -> Saturation/1
  Divide1/1 -> [wcyl]
  [wcyl] -> Data Type Conversion17/1
  Data Type Conversion17/1 -> ctrl_rb_explicit_20131031_v2/9(wcyl)
  ctrl_rb_explicit_20131031_v2/18(egr_rate_est) -> Data Type Conversion23/1
  ctrl_rb_explicit_20131031_v2/19(wegr) -> Data Type Conversion24/1
  Data Type Conversion24/1 -> Terminator_2/1
  Data Type Conversion23/1 -> Terminator_10/1
  Saturation/1 -> Divide1/2
  In1/1 -> Saturation2/1
  Demux/1 -> [fuel_mm3perst]
  Demux/2 -> [engine_speed_rpm]
  In2/1 -> Saturation3/1
  Manual Switch1/1 -> Demux/1
  Mux4/1 -> Manual Switch1/1
  Sum3/1 -> Scope2/1, Out1/1
  Saturation2/1 -> Mux4/1
  Saturation3/1 -> Mux4/2

== system KD_cl_harness_forthao/Combsution ==
  note: W_engine = W_cyl + u_fuel
  note: Gain block has no significance
      | just to add color to the lines
  Omega_engine_radS : Inport
  intake_man_out : Inport  Port=2
  exhaust_man_out : Inport  Port=3
  controls_in : Inport  Port=4
  Bus Creator : BusCreator
  Bus Creator1 : BusCreator
  Bus Selector : BusSelector  OutputSignals=controls_in.u_fuel,omega_engine_data_radS.omega_engine_data_radS,intake_man_out.p_in_man,exhaust_man_out.p_exh_man,intake_man_out.T_in_man,exhaust_man_out.T_exh_man
  Bus Selector1 : BusSelector  OutputSignals=controls_in.u_fuel,intake_man_out.F_in_man
  Bus Selector2 : BusSelector  OutputSignals=omega_engine_data_radS.omega_engine_data_radS,intake_man_out.T_in_man,controls_in.u_fuel,intake_man_out.F_in_man
  "Exhaust " : Subsystem
  Fcn : Fcn  Expr=(u(2)*u(3)+(1+14.6)*u(1))/(u(1)+u(3))
  Gain : Gain
  Mux : Mux  Inputs=3
  Saturation : Saturate  UpperLimit=1  LowerLimit=0
  Sum : Sum
  cylinder comp : Subsystem
  combustion_out : Outport
  W_cyl_sim : Outport  Port=2
  T_exhaust : Outport  Port=3
  W_engine_out : Outport  Port=4
  F_engine_out : Outport  Port=5
  wires:
  cylinder comp/1(W_cyl_sim) -> Gain/1  "W_cylinderr"
  "Exhaust "/1(T_exhaust) -> T_exhaust/1, Bus Creator/2  "T_exhaust"
  Bus Creator/1 -> combustion_out/1  "combustion_out"
  Omega_engine_radS/1 -> Bus Creator1/1
  intake_man_out/1 -> Bus Creator1/2
  exhaust_man_out/1 -> Bus Creator1/3
  controls_in/1 -> Bus Creator1/4
  Bus Creator1/1 -> Bus Selector/1, Bus Selector2/1, Bus Selector1/1
  Bus Selector/2 -> cylinder comp/1(omega_engine_radS)  "<omega_engine_data_radS>"
  Bus Selector/3 -> cylinder comp/2(p_intake_man)  "<p_in_man>"
  Bus Selector/4 -> cylinder comp/3(p_exhaust_man)  "<p_exh_man>"
  Bus Selector/5 -> cylinder comp/4(T_intake_man)  "<T_in_man>"
  Bus Selector/6 -> cylinder comp/5(T_exhaust_man)  "<T_exh_man>"
  Bus Selector2/1 -> "Exhaust "/1(omega_engine_radS)  "<omega_engine_data_radS>"
  Bus Selector2/3 -> "Exhaust "/4(u_fuel)  "<u_fuel>"
  Bus Selector2/4 -> "Exhaust "/5(F1_in_man)  "<F_in_man>"
  Bus Selector2/2 -> "Exhaust "/2(T_intake_man)  "<T_in_man>"
  Bus Selector/1 -> Sum/1  "<u_fuel>"
  Sum/1 -> W_engine_out/1, Bus Creator/4  "W_engine_out"
  Bus Selector1/1 -> Mux/1  "<u_fuel>"
  Bus Selector1/2 -> Mux/2  "<F_in_man>"
  Gain/1 -> "Exhaust "/3(W_cyl), Mux/3, Bus Creator/1, W_cyl_sim/1, Sum/2  "W_cylinder"
  Mux/1 -> Fcn/1
  Fcn/1 -> Saturation/1  "F_engine_out1"
  Saturation/1 -> F_engine_out/1, Bus Creator/3  "F_engine_out"

== system KD_cl_harness_forthao/Compressor ==
  ambient_in : Inport
  pre_throttle_out : Inport  Port=2
  Omega_turbo_radS : Inport  Port=3
  Bus Creator : BusCreator  Inputs=3
  Bus Creator1 : BusCreator  Inputs=3
  Bus Selector : BusSelector  OutputSignals=ambient_in.p_in_comp_data,pre_throttle_out.p_pre_throttle,ambient_in.T_in_comp_data,Omega_turbo_radS.Omega_turbo_radS
  Comp Map : Subsystem
  compressor_out : Outport
  W_comp_sim : Outport  Port=2
  T_out_comp_sim : Outport  Port=3
  Tq_comp_sim : Outport  Port=4
  wires:
  Comp Map/1(W_comp_sim) -> W_comp_sim/1, Bus Creator/1  "W_compressor"
  Comp Map/2(T_out_comp_sim) -> T_out_comp_sim/1, Bus Creator/2  "T_out_comp_sim"
  Bus Creator/1 -> compressor_out/1  "compressor_out"
  Comp Map/3(Tq_comp) -> Tq_comp_sim/1, Bus Creator/3  "Tq_comp_sim"
  ambient_in/1 -> Bus Creator1/1
  pre_throttle_out/1 -> Bus Creator1/2
  Omega_turbo_radS/1 -> Bus Creator1/3
  Bus Creator1/1 -> Bus Selector/1
  Bus Selector/1 -> Comp Map/1(p_in_comp)  "<p_in_comp_data>"
  Bus Selector/2 -> Comp Map/2(p_out_comp)  "<p_pre_throttle>"
  Bus Selector/3 -> Comp Map/3(T_in_comp_data)  "<T_in_comp_data>"
  Bus Selector/4 -> Comp Map/4(omega_turbo_data_radS)  "<Omega_turbo_radS>"

== system KD_cl_harness_forthao/EGR Throttle ==
  controls_in : Inport
  Omega_engine_radS : Inport  Port=2
  intake_man_out : Inport  Port=3
  intercooler_out : Inport  Port=4
  p_preThrottle : Inport  Port=5
  Bus Creator : BusCreator  Inputs=1
  Bus Creator1 : BusCreator  Inputs=5
  Bus Selector : BusSelector  OutputSignals=controls_in.u_EGR_throttle,omega_engine_data_radS.omega_engine_data_radS,intake_man_out.p_in_man,intercooler_out.T_out_IC,pre_throttle_out.p_pre_throttle
  EGR Throttle : Subsystem
  egr_throttle_out : Outport
  W_EGR_Throttle : Outport  Port=2
  wires:
  EGR Throttle/1(ThrottleFlow_kgpers) -> Bus Creator/1, W_EGR_Throttle/1  "W_EGR_Throttle"
  Bus Creator/1 -> egr_throttle_out/1  "egr_throttle_out"
  controls_in/1 -> Bus Creator1/1
  Omega_engine_radS/1 -> Bus Creator1/2
  intake_man_out/1 -> Bus Creator1/3
  intercooler_out/1 -> Bus Creator1/4
  Bus Creator1/1 -> Bus Selector/1
  Bus Selector/1 -> EGR Throttle/1(u_EGR_throttle)  "<u_EGR_throttle>"
  Bus Selector/2 -> EGR Throttle/2(omega_engine_radS)  "<omega_engine_data_radS>"
  Bus Selector/3 -> EGR Throttle/3(p_intake_man)  "<p_in_man>"
  Bus Selector/4 -> EGR Throttle/4(T_out_IC)  "<T_out_IC>"
  Bus Selector/5 -> EGR Throttle/5(p_preThrottle)  "<p_pre_throttle>"
  p_preThrottle/1 -> Bus Creator1/5

== system KD_cl_harness_forthao/EGR Valve ==
  controls_in : Inport
  omega_engine_data_radS : Inport  Port=2
  intake_man_out : Inport  Port=3
  exhaust_man_out : Inport  Port=4
  egr_cooler_out : Inport  Port=5
  Bus Creator : BusCreator  Inputs=1
  Bus Creator1 : BusCreator  Inputs=5
  Bus Selector : BusSelector  OutputSignals=controls_in.u_EGR_valve,omega_engine_data_radS.omega_engine_data_radS,intake_man_out.p_in_man,egr_cooler_out.T_out_EGR_cooler,exhaust_man_out.p_exh_man
  SVR EGR : Subsystem
  egr_valve_out : Outport
  W_EGR_out : Outport  Port=2
  wires:
  SVR EGR/1(EGR_kgpers) -> Bus Creator/1, W_EGR_out/1  "W_EGR_valve"
  Bus Creator/1 -> egr_valve_out/1  "egr_valve_out"
  controls_in/1 -> Bus Creator1/1
  omega_engine_data_radS/1 -> Bus Creator1/2
  intake_man_out/1 -> Bus Creator1/3
  exhaust_man_out/1 -> Bus Creator1/4
  Bus Creator1/1 -> Bus Selector/1
  Bus Selector/1 -> SVR EGR/1(u_EGR_valve)  "<u_EGR_valve>"
  Bus Selector/2 -> SVR EGR/2(omega_engine_data_radS)  "<omega_engine_data_radS>"
  Bus Selector/3 -> SVR EGR/3(p_intake_man_data)  "<p_in_man>"
  Bus Selector/4 -> SVR EGR/4(T_out_egr_cooler)  "<T_out_EGR_cooler>"
  Bus Selector/5 -> SVR EGR/5(p_exhaust_man_data)  "<p_exh_man>"
  egr_cooler_out/1 -> Bus Creator1/5

== system KD_cl_harness_forthao/EGR cooler ==
  note: Estimation of T_in_egr cooler is to be done
      | as T_exh_man and T_in_egr_cooler are
      | significantly different
  T_exh_man : Inport
  ambient_in : Inport  Port=2
  egr_valve_out : Inport  Port=3
  controls_in : Inport  Port=4
  Omega_engine_radS : Inport  Port=5
  Bus Creator : BusCreator  Inputs=2
  Bus Creator1 : BusCreator  Inputs=5
  Bus Selector : BusSelector  OutputSignals=exhaust_man_out.T_exh_man,ambient_in.T_coolant,egr_valve_out.W_EGR_valve,controls_in.u_EGR_cooler_bypass,omega_engine_data_radS.omega_engine_data_radS,ambient_in.T_ambient
  EGR Cooler : Subsystem
  egr_cooler_out : Outport
  T_out_EGR_cooler : Outport  Port=2
  wires:
  EGR Cooler/1(T_out_EGR_cooler_sim) -> Bus Creator/1, T_out_EGR_cooler/1  "T_out_EGR_cooler"
  Bus Creator/1 -> egr_cooler_out/1  "egr_cooler_out"
  Bus Creator1/1 -> Bus Selector/1
  Bus Selector/1 -> EGR Cooler/1(T_exh_man)  "<T_exh_man>"
  Bus Selector/2 -> EGR Cooler/2(T_coolant)  "<T_coolant>"
  Bus Selector/3 -> EGR Cooler/3(W_egr_valve)  "<W_EGR_valve>"
  Bus Selector/4 -> EGR Cooler/4(u_EGR_cooler_bypass)  "<u_EGR_cooler_bypass>"
  Bus Selector/5 -> EGR Cooler/5(omega_engine_data_radS)  "<omega_engine_data_radS>"
  EGR Cooler/2(W_egr_cooler) -> Bus Creator/2  "W_egr_cooler"
  Bus Selector/6 -> EGR Cooler/6(T_ambient)  "<T_ambient>"
  T_exh_man/1 -> Bus Creator1/1
  ambient_in/1 -> Bus Creator1/2
  egr_valve_out/1 -> Bus Creator1/3
  controls_in/1 -> Bus Creator1/4
  Omega_engine_radS/1 -> Bus Creator1/5

== system KD_cl_harness_forthao/Exhaust Manifold ==
  egr_valve_out : Inport
  controls_in : Inport  Port=2
  turbine_out : Inport  Port=3
  combustion_out : Inport  Port=4
  intake_man_out : Inport  Port=5
  ambient_in : Inport  Port=6
  Bus Creator : BusCreator  Inputs=3
  Bus Creator1 : BusCreator  Inputs=6
  Bus Selector : BusSelector  OutputSignals=egr_valve_out.W_EGR_valve,combustion_out.W_cylinder,controls_in.u_fuel,turbine_out.W_turbine,combustion_out.F_engine_out,combustion_out.T_exhaust,intake_man_out.T_in_man,ambient_in.T_ambient
  Exhaust Manifold : Subsystem
  exhaust_man_out : Outport
  p_exh_man_sim : Outport  Port=2
  T_exh_man_sim : Outport  Port=3
  F_exh_man_sim : Outport  Port=4
  wires:
  Exhaust Manifold/1(p_exh_man_sim) -> p_exh_man_sim/1, Bus Creator/1  "p_exh_man"
  Exhaust Manifold/2(T_exh_man_sim) -> T_exh_man_sim/1, Bus Creator/2  "T_exh_man"
  Exhaust Manifold/3(F_exh_man_sim) -> F_exh_man_sim/1, Bus Creator/3  "F_exh_man"
  Bus Creator/1 -> exhaust_man_out/1  "exhaust_man_out"
  Bus Creator1/1 -> Bus Selector/1
  Bus Selector/3 -> Exhaust Manifold/3(u_fuel)  "<u_fuel>"
  Bus Selector/4 -> Exhaust Manifold/4(W_turbine)  "<W_turbine>"
  Bus Selector/5 -> Exhaust Manifold/5(F_engine_out)  "<F_engine_out>"
  Bus Selector/6 -> Exhaust Manifold/6(exhaust_temp)  "<T_exhaust>"
  egr_valve_out/1 -> Bus Creator1/1
  controls_in/1 -> Bus Creator1/2
  turbine_out/1 -> Bus Creator1/3
  combustion_out/1 -> Bus Creator1/4
  Bus Selector/1 -> Exhaust Manifold/1(W_egr_valve)  "<W_EGR_valve>"
  Bus Selector/2 -> Exhaust Manifold/2(W_cylinder)  "<W_cylinder>"
  intake_man_out/1 -> Bus Creator1/5
  Bus Selector/7 -> Exhaust Manifold/7(T_intake_man)  "<T_in_man>"
  ambient_in/1 -> Bus Creator1/6
  Bus Selector/8 -> Exhaust Manifold/8(T_ambient)  "<T_ambient>"

== system KD_cl_harness_forthao/Intake Manifold ==
  throttle_out : Inport
  egr_cooler_out : Inport  Port=2
  exhaust_man_out : Inport  Port=3
  intecooler_out : Inport  Port=4
  combustion_out : Inport  Port=5
  Bus Creator : BusCreator  Inputs=3
  Bus Creator1 : BusCreator  Inputs=5
  Bus Selector : BusSelector  OutputSignals=egr_throttle_out.W_EGR_Throttle,egr_cooler_out.W_egr_cooler,combustion_out.W_cylinder,exhaust_man_out.F_exh_man,egr_cooler_out.T_out_EGR_cooler,intercooler_out.T_out_IC
  Intake_manifold : Subsystem
  intake_man_out : Outport
  p_in_man_sim : Outport  Port=2
  T_in_man_sim : Outport  Port=3
  F_in_man_sim : Outport  Port=4
  wires:
  Intake_manifold/1(p_in_man_sim) -> p_in_man_sim/1, Bus Creator/1  "p_in_man"
  Intake_manifold/2(T_in_man_sim) -> T_in_man_sim/1, Bus Creator/2  "T_in_man"
  Intake_manifold/3(F_in_man_sim) -> F_in_man_sim/1, Bus Creator/3  "F_in_man"
  Bus Creator/1 -> intake_man_out/1  "intake_man_out"
  throttle_out/1 -> Bus Creator1/1
  egr_cooler_out/1 -> Bus Creator1/2
  exhaust_man_out/1 -> Bus Creator1/3
  Bus Creator1/1 -> Bus Selector/1
  Bus Selector/1 -> Intake_manifold/1(W_throttle)  "<W_EGR_Throttle>"
  Bus Selector/2 -> Intake_manifold/2(W_egr_valve)  "<W_egr_cooler>"
  Bus Selector/4 -> Intake_manifold/4(F2_exhaust_sim)  "<F_exh_man>"
  Bus Selector/5 -> Intake_manifold/5(T_out_egr_cooler)  "<T_out_EGR_cooler>"
  intecooler_out/1 -> Bus Creator1/4
  Bus Selector/6 -> Intake_manifold/6(T_out_IC)  "<T_out_IC>"
  combustion_out/1 -> Bus Creator1/5
  Bus Selector/3 -> Intake_manifold/3(W_cyl_in)  "<W_cylinder>"

== system KD_cl_harness_forthao/Intercooler ==
  compressor_out : Inport
  pre_throttle_out : Inport  Port=2
  T_ambient : Inport  Port=3
  Bus Creator : BusCreator  Inputs=3
  Bus Creator1 : BusCreator  Inputs=2
  Bus Selector : BusSelector  OutputSignals=compressor_out.T_out_comp_sim,pre_throttle_out.p_pre_throttle,ambient_in.T_ambient
  Intercooler : Subsystem
  intercooler_out : Outport
  T_out_IC : Outport  Port=2
  wires:
  compressor_out/1 -> Bus Creator/1
  pre_throttle_out/1 -> Bus Creator/2
  Bus Creator/1 -> Bus Selector/1
  Bus Selector/1 -> Intercooler/1(T_out_comp)  "<T_out_comp_sim>"
  Bus Selector/2 -> Intercooler/2(p_out_comp)  "<p_pre_throttle>"
  Intercooler/1(T_out_IC) -> Bus Creator1/1, T_out_IC/1  "T_out_IC"
  Intercooler/2(p_out_IC) -> Bus Creator1/2  "p_out_IC"
  Bus Creator1/1 -> intercooler_out/1  "intercooler_out"
  T_ambient/1 -> Bus Creator/3
  Bus Selector/3 -> Intercooler/3(T_ambient)  "<T_ambient>"

== system KD_cl_harness_forthao/NEDC_cycle ==
  From Workspace1 : FromWorkspace  VariableName=[ECUTIME s2g_eqfine_eqfine]  SampleTime=sample_time  Interpolate=off  OutputAfterFinalValue=Holding final value
  From Workspace3 : FromWorkspace  VariableName=[ECUTIME s2g_ene_ene]  SampleTime=sample_time  Interpolate=off  OutputAfterFinalValue=Holding final value
  Mux3 : Mux  Inputs=2
  Saturation : Saturate  UpperLimit=inf  LowerLimit=750
      settings: AttributesFormatString=%<LowerLimit>\n%<UpperLimit>
  Saturation1 : Saturate  UpperLimit=inf  LowerLimit=0
      settings: AttributesFormatString=%<LowerLimit>\n%<UpperLimit>
  Out1 : Outport
  wires:
  From Workspace3/1 -> Saturation/1
  From Workspace1/1 -> Saturation1/1
  Saturation1/1 -> Mux3/1
  Saturation/1 -> Mux3/2
  Mux3/1 -> Out1/1

== system KD_cl_harness_forthao/Turbine ==
  omega_turbo_radS : Inport
  exhaust_man_out : Inport  Port=2
  ambient_In : Inport  Port=3
  controls_In : Inport  Port=4
  Bus Creator : BusCreator  Inputs=3
  Bus Creator1 : BusCreator
  Bus Selector : BusSelector  OutputSignals=Omega_turbo_radS.Omega_turbo_radS,exhaust_man_out.p_exh_man,ambient_in.T_ambient,exhaust_man_out.T_exh_man,controls_in.u_VGT
  TurbineMap : Subsystem
  turbine_out : Outport
  W_out_turb_sim : Outport  Port=2
  T_out_turb_sim : Outport  Port=3
  Tq_turbine : Outport  Port=4
  wires:
  TurbineMap/1(W_out_turb_sim) -> W_out_turb_sim/1, Bus Creator/1  "W_turbine"
  TurbineMap/2(T_out_turb_sim) -> T_out_turb_sim/1, Bus Creator/2  "T_out_turbine"
  Bus Creator/1 -> turbine_out/1  "turbine_out"
  TurbineMap/3(Tq_turbine) -> Tq_turbine/1, Bus Creator/3  "Tq_turbine"
  omega_turbo_radS/1 -> Bus Creator1/1
  exhaust_man_out/1 -> Bus Creator1/2
  ambient_In/1 -> Bus Creator1/3
  controls_In/1 -> Bus Creator1/4
  Bus Creator1/1 -> Bus Selector/1
  Bus Selector/3 -> TurbineMap/3(T_ambient)  "<T_ambient>"
  Bus Selector/4 -> TurbineMap/4(T_exhaust_man)  "<T_exh_man>"
  Bus Selector/5 -> TurbineMap/5(u_VGT)  "<u_VGT>"
  Bus Selector/1 -> TurbineMap/1(omega_turbo_radS)  "<Omega_turbo_radS>"
  Bus Selector/2 -> TurbineMap/2(p_exhaust_man)  "<p_exh_man>"

== system KD_cl_harness_forthao/Turbo Rotational Dynamics ==
  compressor_out : Inport
  turbine_out : Inport  Port=2
  Bus Creator : BusCreator  Inputs=1
  Bus Creator1 : BusCreator  Inputs=2
  Bus Selector : BusSelector  OutputSignals=compressor_out.Tq_comp_sim,turbine_out.Tq_turbine
  Turbo rot : Subsystem
  Omega_turbo_radS : Outport
  Omega_turbo_out_radS : Outport  Port=2
  wires:
  Turbo rot/1(Omega_turbo_radS) -> Omega_turbo_out_radS/1, Bus Creator/1  "Omega_turbo_radS"
  Bus Creator/1 -> Omega_turbo_radS/1  "Omega_turbo_radS"
  compressor_out/1 -> Bus Creator1/1
  turbine_out/1 -> Bus Creator1/2
  Bus Creator1/1 -> Bus Selector/1
  Bus Selector/1 -> Turbo rot/1(Tq_compressor)  "<Tq_comp_sim>"
  Bus Selector/2 -> Turbo rot/2(Tq_turbine)  "<Tq_turbine>"

== system KD_cl_harness_forthao/ambient_and_controls_in ==
  Bus Creator1 : BusCreator  Inputs=6
  From Workspace11 : FromWorkspace  VariableName="[0   97.4216]"  SampleTime=0  Interpolate=off  OutputAfterFinalValue=Holding final value
  From Workspace12 : FromWorkspace  VariableName="[0  296.9595]"  SampleTime=0  Interpolate=off  OutputAfterFinalValue=Holding final value
  From Workspace5 : FromWorkspace  VariableName="[0   97.4450]"  SampleTime=0  Interpolate=off  OutputAfterFinalValue=Holding final value
  From Workspace6 : FromWorkspace  VariableName="[0  300.0250]"  SampleTime=0  Interpolate=off  OutputAfterFinalValue=Holding final value
  From Workspace7 : FromWorkspace  VariableName="[0  351.4714]"  SampleTime=0  Interpolate=off  OutputAfterFinalValue=Holding final value
  From Workspace8 : FromWorkspace  VariableName="[0    3.7702]"  SampleTime=0  Interpolate=off  OutputAfterFinalValue=Holding final value
  ambient_in : Outport
  wires:
  Bus Creator1/1 -> ambient_in/1  "ambient_in"
  From Workspace11/1 -> Bus Creator1/1  "p_in_comp_data"
  From Workspace5/1 -> Bus Creator1/2  "p_ambient"
  From Workspace12/1 -> Bus Creator1/3  "T_in_comp_data"
  From Workspace6/1 -> Bus Creator1/4  "T_ambient"
  From Workspace7/1 -> Bus Creator1/5  "T_coolant"
  From Workspace8/1 -> Bus Creator1/6  "Tq_load"
